simulink model "ej6"  (R2023a)
settings: Solver=VariableStepAuto  StartTime=0.0  StopTime=10.0  RelTol=1e-3
model workspace (MAT data in the model file):
  B = 0.1
  g = 0.5
  x0 = 70
settings Model: Creator=santi  LastModifiedBy=santi

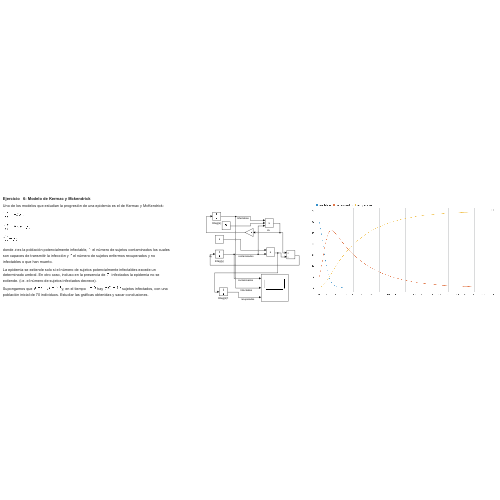
[thumbnail: Simulink's stored preview of the top-level diagram]
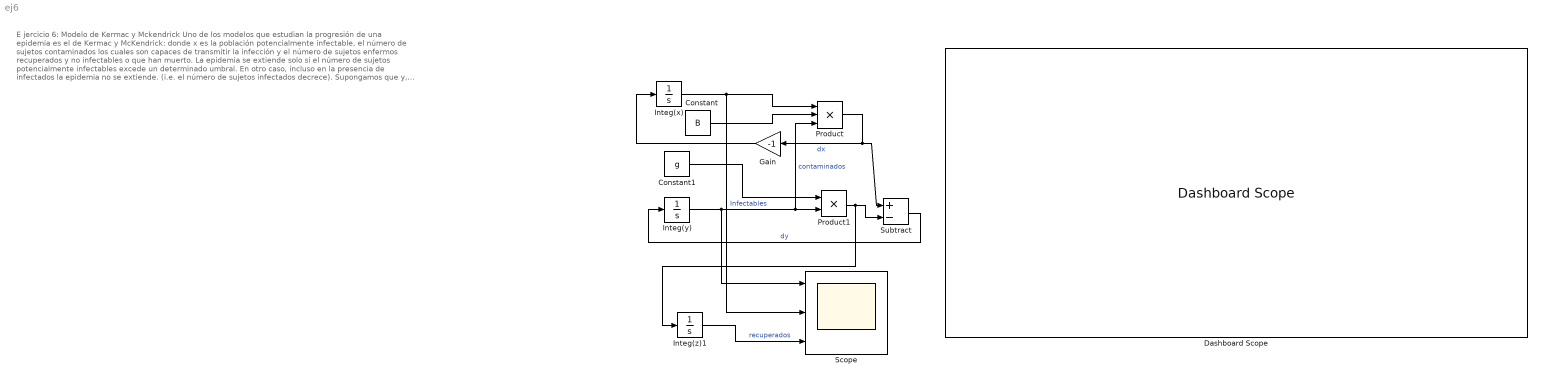
== system ej6 ==
  note: E jercicio 6: Modelo de Kermac y Mckendrick
      | Uno de los modelos que estudian la progresión de una epidemia es el de Kermac y McKendrick:
      |
      | donde x es la población potencialmente infectable, el número de sujetos contaminados los cuales son capaces de transmitir la infección y el número de sujetos enfermos recuperados y no infectables o que han muerto.
      | La epidemia se extiende solo si el número de sujetos potencialmente infectables excede un determinado umbral. En otro caso, incluso en la presencia de infectados la epidemia no se extiende. (i.e. el número de sujetos infectados decrece).
      | Supongamos que y, en el tiempo hay sujetos infectados, con una población inicial de 70 individuos. Estudiar las gráficas obtenidas y sacar conclusiones.
  Constant : Constant  Value=B
  Constant1 : Constant  Value=g
  Dashboard Scope : DashboardScope
  Gain : Gain  Gain=-1
  Integ(x) : Integrator  InitialCondition=60
  Integ(y) : Integrator  InitialCondition=10
  Integ(z)1 : Integrator
  Product : Product  Inputs=3
  Product1 : Product
  Scope : Scope  NumInputPorts=3
  Subtract : Sum  Inputs=+-
  wires:
  Integ(x)/1 -> Scope/2, Product/1  "Infectables"
  Product/1 -> Gain/1, Subtract/1  "dx"
  Subtract/1 -> Integ(y)/1  "dy"
  Integ(y)/1 -> Scope/1, Product1/2, Product/3  "contaminados"
  Constant/1 -> Product/2
  Gain/1 -> Integ(x)/1
  Constant1/1 -> Product1/1
  Product1/1 -> Integ(z)1/1, Subtract/2
  Integ(z)1/1 -> Scope/3  "recuperados"
